simulink model "revision"  (R2019b)
settings: Solver=VariableStepAuto  StartTime=0.0  StopTime=10.0  RelTol=1e-3
libraries: commfilt2 x2, commsink2 x1, commutil2 x1, commrandsrc3 x1
settings Model: Creator=DELL  LastModifiedBy=DELL

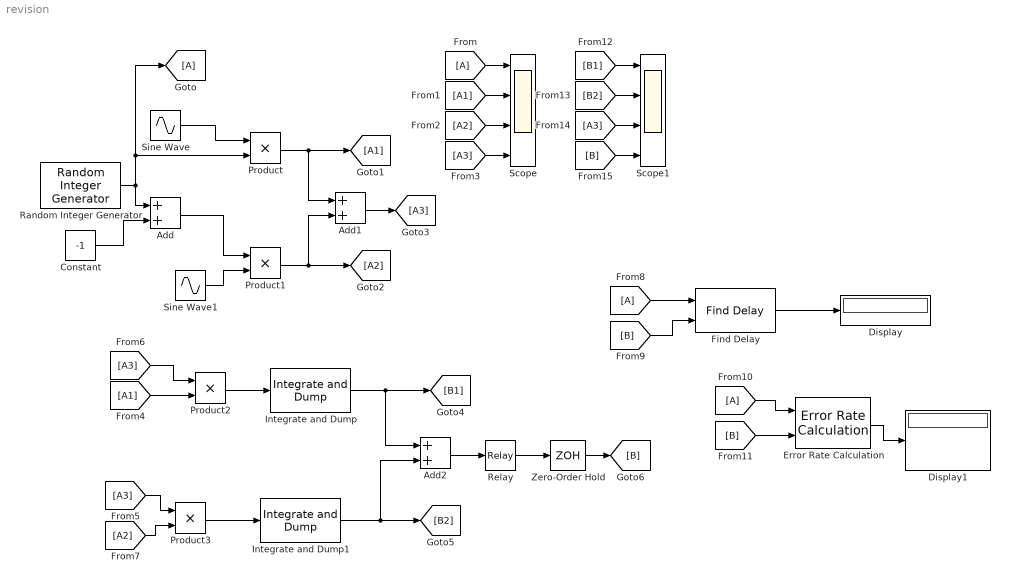
== system revision ==
  Add : Sum
  Add1 : Sum
  Add2 : Sum
  Constant : Constant  Value=-1
  Display : Display
  Display1 : Display
  Error Rate Calculation : commsink2/Error Rate Calculation  N=1  st_delay=0  cp_mode=Entire frame  subframe=[]  PMode=Port  WsName=ErrorVec  RsMode2=off  stop=off  numErr=100  maxBits=1e6
      settings: SourceProductName=Communications Toolbox
  Find Delay : commutil2/Find Delay  corrLength=200  chgSigOP=off  stopUpdate=off  numConstDelay=3
      settings: SourceProductName=Communications Toolbox  SourceProductBaseCode=CM
  Integrate and Dump : commfilt2/Integrate and Dump  obssamples=100  offsetsamples=0  nodump=off  roundingMode=Floor  overflowMode=off  outputDataTypeStr=Inherit: Same as accumulator  outputLastDataTypeStr=Inherit: Same as accumulator
      settings: SourceProductName=Communications Toolbox
  Integrate and Dump1 : commfilt2/Integrate and Dump  obssamples=100  offsetsamples=0  nodump=off  roundingMode=Floor  overflowMode=off  outputDataTypeStr=Inherit: Same as accumulator  outputLastDataTypeStr=Inherit: Same as accumulator
      settings: SourceProductName=Communications Toolbox
  Product{,1..3} (4 alike) : Product
  Random Integer Generator : commrandsrc3/Random Integer Generator  SetSize=2  SeedSource=Auto  Seed=0  SampleTime=1/1000  SamplesPerFrame=1  OutputDataType=double  SimulateUsing=Interpreted execution
      settings: SourceProductName=Communications Toolbox
  Relay : Relay  OnSwitchValue=0  OffSwitchValue=0
  Scope : Scope  NumInputPorts=4
  Scope1 : Scope  NumInputPorts=4
  Sine Wave : Sin  Frequency=2*pi*10000  SampleTime=1/100000
  Sine Wave1 : Sin  Frequency=2*pi*11000  SampleTime=1/100000
  Zero-Order Hold : ZeroOrderHold  SampleTime=1/1000
  wires:
  Random Integer Generator/1 -> [A], Product/2, Add/1
  Constant/1 -> Add/2
  Add/1 -> Product1/1
  Sine Wave1/1 -> Product1/2
  Sine Wave/1 -> Product/1
  Product/1 -> [A1], Add1/1
  Product1/1 -> [A2], Add1/2
  Add1/1 -> [A3]
  [A] -> Scope/1
  [A1] -> Scope/2
  [A2] -> Scope/3
  [A3] -> Scope/4
  Product2/1 -> Integrate and Dump/1
  Product3/1 -> Integrate and Dump1/1
  [A3] -> Product3/1
  [A2] -> Product3/2
  Integrate and Dump/1 -> [B1], Add2/1
  Integrate and Dump1/1 -> [B2], Add2/2
  Add2/1 -> Relay/1
  Relay/1 -> Zero-Order Hold/1
  Zero-Order Hold/1 -> [B]
  [A] -> Find Delay/1
  [B] -> Find Delay/2
  [A] -> Error Rate Calculation/1
  [B] -> Error Rate Calculation/2
  Find Delay/1 -> Display/1
  Error Rate Calculation/1 -> Display1/1
  [B] -> Scope1/4
  [A3] -> Scope1/3
  [B2] -> Scope1/2
  [B1] -> Scope1/1
  [A1] -> Product2/2
  [A3] -> Product2/1
